simulink subsystem "Decay_Power"  (R2024a)
settings: Solver=VariableStepAuto  StartTime=0.0  StopTime=10.0  RelTol=1e-3
undefined symbols (not defined in the file): coreFuelVolume, outCoreFuelVolume, thermalPower, Volume
libraries: fl_lib x2, nesl_utility x1
settings Model: Creator=silen  LastModifiedBy=silen

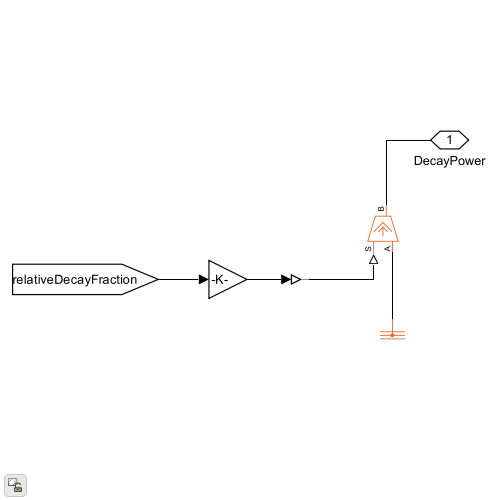
[thumbnail: Simulink's stored preview of the top-level diagram]
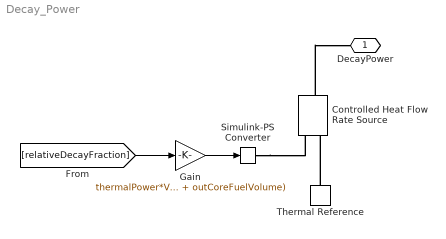
== system Decay_Power ==
  Controlled Heat Flow Rate Source : fl_lib/Thermal/Thermal Sources/Controlled Heat Flow Rate Source
  Gain : Gain  Gain=thermalPower*Volume./(coreFuelVolume + outCoreFuelVolume)
  Simulink-PS Converter : nesl_utility/Simulink-PS Converter  PhysicalDomain=network_engine_domain  SubClassName=ps_input  LeftPortType=input  RightPortType=output  PseudoPeriodic=off  Frequencies=[]  NoiseDistribution=none  NoiseParameters=[]  Unit=W  AffineConversion=off  FilteringAndDerivatives=provide  SimscapeFilterOrder=1  InputFilterTimeConstant=0.001  UdotUserProvided=0
  Thermal Reference : fl_lib/Thermal/Thermal Elements/Thermal Reference
  DecayPower : PMIOPort  Side=Left
  wires:
  [relativeDecayFraction] -> Gain/1
  Gain/1 -> Simulink-PS Converter/1
  connections:
  Controlled Heat Flow Rate Source/LConn1 -- DecayPower/RConn1
  Simulink-PS Converter/RConn1 -- Controlled Heat Flow Rate Source/RConn1
  Thermal Reference/LConn1 -- Controlled Heat Flow Rate Source/RConn2
